simulink model "RudderActuatorChannel_control_arx"  (R2015a)
settings: Solver=ode4  StartTime=0.0  StopTime=2.999  FixedStep=sampleTime  MaxStep=1e-3  MinStep=1e-4
undefined symbols (not defined in the file or in its folder): Acv, Aleak1, Aleak2, Aleak3, Aleak4, Aleak5, Aleakext, Aleakint, Ap, Ap_seal, Ar_seal, As_ehsv, Bkp_seal, Bp1, C, Cd, ControlTopology, DeltaQ_ehsv, EHSV, EHSV_Step, EHSVFreqTest, EHSVTest, ent_air, frictionstribeck_velocity, i_ehsv, Imax, K2_ehsv, K3_ehsv, K_Supply1, Ka1, Kd, Ki, Ki_ehsv, Kp, Kr_ehsv, ksi_ehsv, Kst, Kst_Enable, Kw_ehsv, L0, Load_cmd, Lp_seal, Lr_seal, Max_Cmd, Max_Load_TED, Max_Load_TEU, Min_Cmd, Mp1, ON_OFF_hyst, P10, Pcvac, Pcvi, Pcvr, Ps0, Pt0, Ql_ehsv, R, Rate_Limit, Return_Pressure, Rho ... (+24)
undefined symbols (not defined in the file): dpLVDT, Kd_N, ramLVDT, StateControl, xvLVDT
libraries: simulink x3
(part 1 of 2)
settings Model: SimulationMode=accelerator  Creator=Charles  LastModifiedBy=Pedro H
settings SolverCC: InitialStep=1e-4
settings DataIOCC: LimitDataPoints=off  SaveFormat=StructureWithTime  DSMLogging=off  SaveTime=off
settings OptimizationCC: ExpressionDepthLimit=2147483647  InitFltsAndDblsToZero=on
settings DebuggingCC: SaveWithParameterizedLinksMsg=none  UnderspecifiedInitializationDetection=Classic  MergeDetectMultiDrivingBlocksExec=none  SolverPrmCheckMsg=warning  InheritedTsInSrcMsg=none  FcnCallInpInsideContextMsg=UseLocalSettings  StateNameClashWarn=warning
settings ModelReferenceCC: UpdateModelReferenceTargets=IfOutOfDate
settings GRTTargetCC: TargetFcnLib=ansi_tfl_tmw.mat  CombineOutputUpdateFcns=off  GRTInterface=on

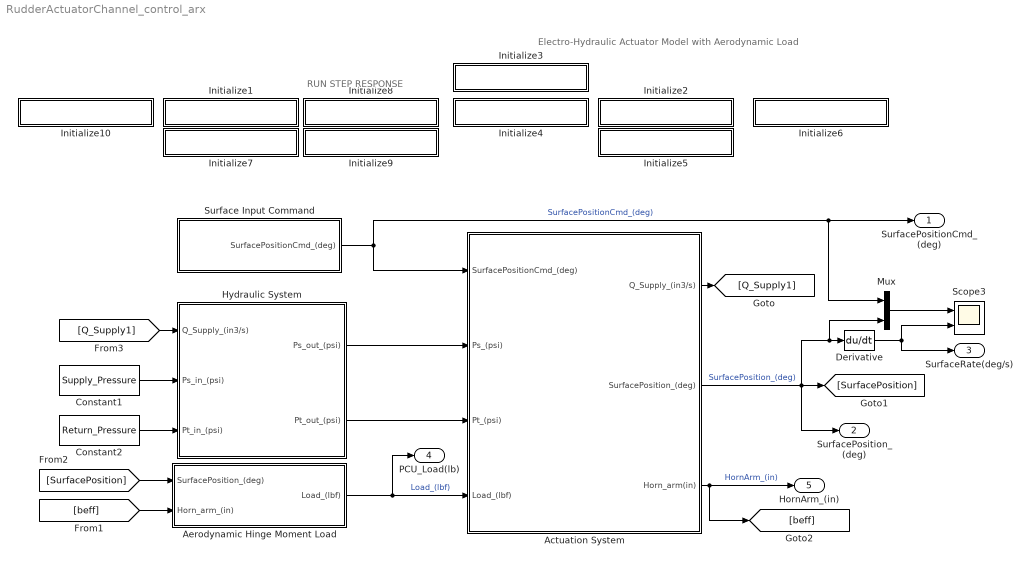
== system RudderActuatorChannel_control_arx ==
  note: RUN STEP RESPONSE
  note: Electro-Hydraulic Actuator Model with Aerodynamic Load
  Actuation System : Subsystem
  Aerodynamic Hinge Moment Load : Subsystem
  Constant1 : Constant  Value=Supply_Pressure
  Constant2 : Constant  Value=Return_Pressure
  Derivative : Derivative  CoefficientInTFapproximation=1e6
  Hydraulic System : Subsystem
  Initialize1 : Subsystem
      settings: OpenFcn=|
      | run('StepInput_CLLoad.m'),
      | set_param(bdroot,'SimulationCommand','start')
      mask Display: disp('Closed Loop - Loaded')
  Initialize10 : Subsystem
      settings: OpenFcn=|
      | run('SineInput_CLLoad.m'),
      | set_param(bdroot,'SimulationCommand','start')
      mask Display: disp('Run Sine Input')
  Initialize2 : Subsystem
      settings: OpenFcn=|
      | FreqResp_type = 0;
      | run('FrequencyResponseTest.m'),
      | set_param(bdroot,'SimulationCommand','start')
      mask Display: disp('Frequency Response')
  Initialize3 : Subsystem
      settings: OpenFcn=run('Load_Parameters.m'),
      mask Display: disp('Model Initialization')
  Initialize4 : Subsystem
      settings: OpenFcn=run('plotMaster.m')
      mask Display: disp('Plot Results')
  Initialize5 : Subsystem
      settings: OpenFcn=|
      | FreqResp_type = 1;
      | run('FrequencyResponseTest.m'),
      | set_param(bdroot,'SimulationCommand','start')
      mask Display: disp('Run EHSV Frequency Response Test')
  Initialize6 : Subsystem
      settings: OpenFcn=run('DynamicStiffnessTest.m')
      mask Display: disp('Dynamic Stiffness Test')
  Initialize7 : Subsystem
      settings: OpenFcn=|
      | run('StepInput_CLNoLoad.m'),
      | set_param(bdroot,'SimulationCommand','start')
      mask Display: disp('Closed Loop - Unloaded')
  Initialize8 : Subsystem
      settings: OpenFcn=|
      | run('StepInput_OLEHSVLoad.m'),
      | set_param(bdroot,'SimulationCommand','start')
      mask Display: disp('Open Loop - Loaded')
  Initialize9 : Subsystem
      settings: OpenFcn=|
      | run('StepInput_OLEHSVNoLoad.m'),
      | set_param(bdroot,'SimulationCommand','start')
      mask Display: disp('Open Loop - Unloaded')
  Mux : Mux  Inputs=2
  Scope3 : Scope  NumInputPorts=2
      settings: TimeRange=3.4  YMin=28.7~-5  YMax=30.8~5  SaveName=Theta
  Surface Input Command : Subsystem
  SurfacePositionCmd_(deg) : Outport
  SurfacePosition_(deg) : Outport  Port=2
  SurfaceRate(deg/s) : Outport  Port=3
  PCU_Load(lb) : Outport  Port=4
  HornArm_(in) : Outport  Port=5
  wires:
  Constant1/1 -> Hydraulic System/2(Ps_in_(psi))
  Constant2/1 -> Hydraulic System/3(Pt_in_(psi))
  Hydraulic System/1(Ps_out_(psi)) -> Actuation System/2(Ps_(psi))
  Hydraulic System/2(Pt_out_(psi)) -> Actuation System/3(Pt_(psi))
  Actuation System/1(Q_Supply_(in3/s)) -> [Q_Supply1]
  [Q_Supply1] -> Hydraulic System/1(Q_Supply_(in3/s))
  Actuation System/2(SurfacePosition_(deg)) -> SurfacePosition_(deg)/1, [SurfacePosition], Mux/2, Derivative/1  "SurfacePosition_(deg)"
  [SurfacePosition] -> Aerodynamic Hinge Moment Load/1(SurfacePosition_(deg))
  Surface Input Command/1(SurfacePositionCmd_(deg)) -> Mux/1, SurfacePositionCmd_(deg)/1, Actuation System/1(SurfacePositionCmd_(deg))  "SurfacePositionCmd_(deg)"
  Actuation System/3(Horn_arm(in)) -> [beff], HornArm_(in)/1  "HornArm_(in)"
  [beff] -> Aerodynamic Hinge Moment Load/2(Horn_arm_(in))
  Aerodynamic Hinge Moment Load/1(Load_(lbf)) -> Actuation System/4(Load_(lbf)), PCU_Load(lb)/1  "Load_(lbf)"
  Derivative/1 -> Scope3/2, SurfaceRate(deg/s)/1
  Mux/1 -> Scope3/1

== system RudderActuatorChannel_control_arx/Actuation System ==
  SurfacePositionCmd_(deg) : Inport
  Ps_(psi) : Inport  Port=2
  Pt_(psi) : Inport  Port=3
  Load_(lbf) : Inport  Port=4
  Actuator : Subsystem
  Bus Creator : BusCreator  Inputs=2
  Electronics System : Subsystem
  Scope : Scope
      settings: SaveName=ScopeData6
  Surface Kinematics : Subsystem
  Q_Supply_(in3/s) : Outport
  SurfacePosition_(deg) : Outport  Port=2
  Horn_arm(in) : Outport  Port=3
  wires:
  [Sensors_FB] -> Electronics System/2(Sensors_FB)
  SurfacePositionCmd_(deg)/1 -> [Theta_Cmd]
  [Theta_Cmd] -> Electronics System/1(Theta_Cmd_(deg))
  Ps_(psi)/1 -> Bus Creator/1  "Ps"
  Pt_(psi)/1 -> Bus Creator/2  "Pt"
  Bus Creator/1 -> Actuator/3(Hyd_Power)
  Actuator/2(Q_Supply) -> Q_Supply_(in3/s)/1
  Actuator/1(Xp_real_(in)) -> Surface Kinematics/1(Xp_(in))  "Xp"
  Load_(lbf)/1 -> [Load]
  Surface Kinematics/1(ThetaPos_(deg)) -> SurfacePosition_(deg)/1
  Actuator/3(Sensors) -> [Sensors_FB]
  Surface Kinematics/2(Effective_arm_(in)) -> Horn_arm(in)/1
  [Load] -> Scope/1, Actuator/2(Load)
  Electronics System/1(Current_Cmd_(mA)) -> Actuator/1(Current_Cmd)

== system RudderActuatorChannel_control_arx/Aerodynamic Hinge Moment Load ==
  note: Aerodynamic Hinge Moment Load
  SurfacePosition_(deg) : Inport
  Horn_arm_(in) : Inport  Port=2
  1-D Lookup Table : Lookup_n-D  NumberOfTableDimensions=1  BreakpointsForDimension1=[-1 0 1]  Table=[-Max_Load_TED 0 Max_Load_TEU]  RndMeth=Simplest  InputSameDT=on
  Constant : Constant  Value=StiffnessTest_Enable
  Constant1 : Constant  Value=Load_cmd
  Divide : Product  Inputs=*/
  Gain : Gain  Gain=1/Max_Cmd
  Load Type Selector : MultiPortSwitch
  Stiffness Test Load : Sin  Amplitude=StiffTest.Sine_Amplitude  Bias=StiffTest.Sine_Bias  Frequency=StiffTest.Sine_Frequency  SampleTime=0
  Load_(lbf) : Outport
  wires:
  SurfacePosition_(deg)/1 -> Gain/1
  Constant/1 -> Load Type Selector/1
  Gain/1 -> 1-D Lookup Table/1
  Load Type Selector/1 -> Load_(lbf)/1
  Stiffness Test Load/1 -> Load Type Selector/2
  Constant1/1 -> Load Type Selector/4
  1-D Lookup Table/1 -> Divide/1
  Divide/1 -> Load Type Selector/3
  Horn_arm_(in)/1 -> Divide/2

== system RudderActuatorChannel_control_arx/Hydraulic System ==
  Q_Supply_(in3/s) : Inport
  Ps_in_(psi) : Inport  Port=2
  Pt_in_(psi) : Inport  Port=3
  Aircraft Hydraulic Losses : Gain  Gain=K_Supply1
  Bus Selector : BusSelector  OutputSignals=Qs
  Fluid Inertia : TransferFcn  Denominator=[0.01 1]
  Sum1 : Sum  Inputs=|+-
  cis to gpm : Gain  Gain=0.25974
  Ps_out_(psi) : Outport
  Pt_out_(psi) : Outport  Port=2
  wires:
  Sum1/1 -> Ps_out_(psi)/1  "Ps"
  Aircraft Hydraulic Losses/1 -> Fluid Inertia/1
  Fluid Inertia/1 -> Sum1/2
  Pt_in_(psi)/1 -> Pt_out_(psi)/1  "Pt"
  Ps_in_(psi)/1 -> Sum1/1  "Ps"
  Q_Supply_(in3/s)/1 -> Bus Selector/1
  cis to gpm/1 -> Aircraft Hydraulic Losses/1
  Bus Selector/1 -> cis to gpm/1  "<Qs>"

== system RudderActuatorChannel_control_arx/Initialize1 ==

== system RudderActuatorChannel_control_arx/Initialize10 ==

== system RudderActuatorChannel_control_arx/Initialize2 ==

== system RudderActuatorChannel_control_arx/Initialize3 ==

== system RudderActuatorChannel_control_arx/Initialize4 ==

== system RudderActuatorChannel_control_arx/Initialize5 ==

== system RudderActuatorChannel_control_arx/Initialize6 ==

== system RudderActuatorChannel_control_arx/Initialize7 ==

== system RudderActuatorChannel_control_arx/Initialize8 ==

== system RudderActuatorChannel_control_arx/Initialize9 ==

== system RudderActuatorChannel_control_arx/Surface Input Command ==
  Repeating Sequence : simulink/Sources/Repeating Sequence  rep_seq_t=[0 0.001 1.5 1.501 3 3.001 4.5 4.501 6 6.001 7.5 7.501 9 9.001 10.5 10.501 12 12.001 13.5 13.501 15]  rep_seq_y=[0 1 1 -1 -1 0.6 0.6 -0.8 -0.8 -0.1 -0.1 0.9 0.9 -0.7 -0.7 0 0 -0.5 -0.5 1 1]
  Repeating Sequence1 : simulink/Sources/Repeating Sequence  rep_seq_t=[0 0.001 1 1.001 2 2.001 3 3.001 4 4.001 5 5.001 6 6.001 7 7.001 8 8.001 9 9.001 10 10.001 11 11.001 12 12.001 13 13.001 14 14.001 15]  rep_seq_y=[0 1 1 1 1 -1 -1 1 1 -1 -1 -1 -1 1 1 1 1 -1 -1 1 1 -1 -1 -1 -1 -1 -1 1 1 1 1]
  SurfacePositionCmd_(deg) : Outport
  wires:
  Repeating Sequence/1 -> SurfacePositionCmd_(deg)/1

== system RudderActuatorChannel_control_arx/Actuation System/Actuator ==
  Current_Cmd : Inport
  Load : Inport  Port=2
  Hyd_Power : Inport  Port=3
  Cylinder Dynamics : Subsystem
  Sensors Dynamics : Subsystem
  Valves Dynamics : Subsystem
  Xp_real_(in) : Outport
  Q_Supply : Outport  Port=2
  Sensors : Outport  Port=3
  wires:
  Cylinder Dynamics/2(Xp) -> [Xp], Xp_real_(in)/1
  Load/1 -> Cylinder Dynamics/2(Load)
  Valves Dynamics/2(Q_Supply) -> Q_Supply/1
  Valves Dynamics/1(Q_Act) -> Cylinder Dynamics/1(Q_Act)
  Current_Cmd/1 -> Valves Dynamics/2(Currrent)
  Hyd_Power/1 -> Valves Dynamics/3(Hyd_Pwr)
  Cylinder Dynamics/1(P_Act) -> Valves Dynamics/1(P_Act)
  Cylinder Dynamics/3(Qacv) -> Valves Dynamics/4(Qacv)
  Valves Dynamics/3(Pt) -> Cylinder Dynamics/3(Pt)
  Valves Dynamics/4(Xv_(in)) -> [Xv]
  Cylinder Dynamics/4(dP) -> [dP]
  [Xp] -> Sensors Dynamics/1(Xp)
  [dP] -> Sensors Dynamics/2(dP)
  [Xv] -> Sensors Dynamics/3(Xv)
  Sensors Dynamics/1(Sensors) -> Sensors/1

== system RudderActuatorChannel_control_arx/Actuation System/Electronics System ==
  Theta_Cmd_(deg) : Inport
  Sensors_FB : Inport  Port=2
  Analog Controller : Subsystem
  Constant : Constant  Value=ControlTopology
  Digital Controller : Subsystem
  Hardware_in : Subsystem
  Hardware_out : Subsystem
  Switch : Switch  Threshold=5.5
  Current_Cmd_(mA) : Outport
  wires:
  Theta_Cmd_(deg)/1 -> Analog Controller/1(Cmd_D), Hardware_in/1(Theta_Cmd_in)
  Digital Controller/1(EHSV_Cmd) -> Hardware_out/1(EHSV_Cmd_in)
  Hardware_out/1(EHSV_Cmd_out) -> Switch/3  "Current_Cmd_CL"
  Hardware_in/1(Theta_Cmd_out) -> Digital Controller/1(Cmd_D)
  Hardware_in/2(Sensors_FB_out) -> Digital Controller/2(Sensors_FB)
  Sensors_FB/1 -> Analog Controller/2(Sensors_FB), Hardware_in/2(Sensors_FB_in)
  Switch/1 -> Current_Cmd_(mA)/1
  Analog Controller/1(EHSV_Cmd) -> Switch/1
  Constant/1 -> Switch/2

== system RudderActuatorChannel_control_arx/Actuation System/Surface Kinematics ==
  Xp_(in) : Inport
  Rad2Deg : Gain  Gain=180/pi  SaturateOnIntegerOverflow=on  OutDataTypeStr=Inherit: Same as input  ParamDataTypeStr=Inherit: Same as input
  Real Kinematics : Subsystem
  ThetaPos_(deg) : Outport
  Effective_arm_(in) : Outport  Port=2
  wires:
  Xp_(in)/1 -> Real Kinematics/1(Xp)
  Real Kinematics/1(Theta) -> Rad2Deg/1
  Rad2Deg/1 -> ThetaPos_(deg)/1
  Real Kinematics/2(Reff) -> Effective_arm_(in)/1

== system RudderActuatorChannel_control_arx/Actuation System/Actuator/Cylinder Dynamics ==
  Q_Act : Inport
  Load : Inport  Port=2
  Pt : Inport  Port=3
  Bus Creator1 : BusCreator  Inputs=2
  Bus Creator3 : BusCreator  Inputs=2
  Bus Selector : BusSelector  OutputSignals=Q1,Q2
  Fluid Dynamics : Subsystem
  Piston Dynamics : Subsystem
  Scope : Scope  NumInputPorts=5
      settings: YMin=-5~-5~-5~-5~-5  YMax=5~5~5~5~5  SaveName=ScopeData8
  P_Act : Outport
  Xp : Outport  Port=2
  Qacv : Outport  Port=3
  dP : Outport  Port=4
  wires:
  Bus Creator3/1 -> P_Act/1
  Q_Act/1 -> Bus Selector/1
  Bus Selector/2 -> Fluid Dynamics/4(Q2)  "<Q2>"
  Piston Dynamics/1(Xp) -> [Xp], Xp/1
  Piston Dynamics/2(Xpdot) -> [Xpdot]  "Xpdot"
  [Xp] -> Scope/3, Fluid Dynamics/1(xp)
  [Xpdot] -> Scope/4, Fluid Dynamics/2(xpdot)
  Load/1 -> Piston Dynamics/3(FL)
  Bus Selector/1 -> Fluid Dynamics/3(Q1)  "<Q1>"
  Fluid Dynamics/2(P2) -> Scope/2, Piston Dynamics/2(Pr), Bus Creator3/2  "P2"
  Fluid Dynamics/1(P1) -> Scope/1, Piston Dynamics/1(Pe), Bus Creator3/1  "P1"
  Pt/1 -> Fluid Dynamics/5(Pt)
  Fluid Dynamics/3(Qacv1) -> Bus Creator1/1  "Qacv1"
  Fluid Dynamics/4(Qacv2) -> Bus Creator1/2  "Qacv2"
  Bus Creator1/1 -> Qacv/1
  Fluid Dynamics/5(dP) -> Scope/5, dP/1

== system RudderActuatorChannel_control_arx/Actuation System/Actuator/Sensors Dynamics ==
  Xp : Inport
  dP : Inport  Port=2
  Xv : Inport  Port=3
  Bus Creator : BusCreator  Inputs=3
  "Xp LVDT " : Subsystem
  "Xv LVDT " : Subsystem
  "dP LVDT " : Subsystem
  Sensors : Outport
  wires:
  dP/1 -> "dP LVDT "/1(dP_real)
  Xp/1 -> "Xp LVDT "/1(Xp_real)
  Xv/1 -> "Xv LVDT "/1(Xv_real)
  "Xv LVDT "/1(Xv_LVDT) -> Bus Creator/3  "Xv_mesured_(in)"
  "dP LVDT "/1(dP_LVDT) -> Bus Creator/2  "dP_mesured_(psi)"
  "Xp LVDT "/1(Xp_LVDT) -> Bus Creator/1  "Xp_mesured_(in)"
  Bus Creator/1 -> Sensors/1

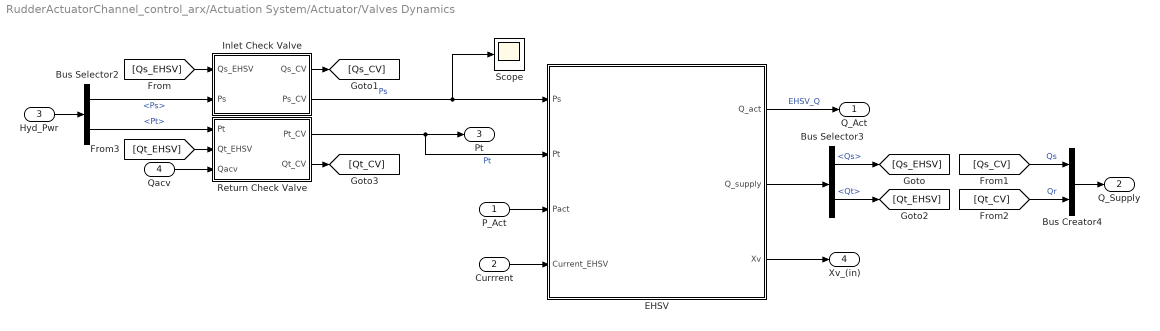
== system RudderActuatorChannel_control_arx/Actuation System/Actuator/Valves Dynamics ==
  P_Act : Inport
  Currrent : Inport  Port=2
  Hyd_Pwr : Inport  Port=3
  Qacv : Inport  Port=4
  Bus Creator4 : BusCreator  Inputs=2
  Bus Selector2 : BusSelector  OutputSignals=Ps,Pt
  Bus Selector3 : BusSelector  OutputSignals=Qs,Qt
  EHSV : Subsystem
  Inlet Check Valve : Subsystem
  Return Check Valve : Subsystem
  Scope : Scope
      settings: SaveName=ScopeData5
  Q_Act : Outport
  Q_Supply : Outport  Port=2
  Pt : Outport  Port=3
  Xv_(in) : Outport  Port=4
  wires:
  Hyd_Pwr/1 -> Bus Selector2/1
  EHSV/1(Q_act) -> Q_Act/1  "EHSV_Q"
  Bus Selector2/1 -> Inlet Check Valve/2(Ps)  "<Ps>"
  Bus Selector3/1 -> [Qs_EHSV]  "<Qs>"
  [Qs_EHSV] -> Inlet Check Valve/1(Qs_EHSV)
  Inlet Check Valve/1(Qs_CV) -> [Qs_CV]
  [Qs_CV] -> Bus Creator4/1  "Qs"
  Bus Creator4/1 -> Q_Supply/1
  Bus Selector2/2 -> Return Check Valve/1(Pt)  "<Pt>"
  Bus Selector3/2 -> [Qt_EHSV]  "<Qt>"
  [Qt_CV] -> Bus Creator4/2  "Qr"
  [Qt_EHSV] -> Return Check Valve/2(Qt_EHSV)
  Return Check Valve/2(Qt_CV) -> [Qt_CV]
  Qacv/1 -> Return Check Valve/3(Qacv)
  Currrent/1 -> EHSV/4(Current_EHSV)
  P_Act/1 -> EHSV/3(Pact)
  Inlet Check Valve/2(Ps_CV) -> Scope/1, EHSV/1(Ps)  "Ps"
  Return Check Valve/1(Pt_CV) -> EHSV/2(Pt), Pt/1  "Pt"
  EHSV/2(Q_supply) -> Bus Selector3/1
  EHSV/3(Xv) -> Xv_(in)/1

== system RudderActuatorChannel_control_arx/Actuation System/Electronics System/Analog Controller ==
  Cmd_D : Inport
  Sensors_FB : Inport  Port=2
  Command Limits : Saturate  UpperLimit=Max_Cmd  LowerLimit=Min_Cmd
  Deg2Rad : Gain  Gain=pi/180  SaturateOnIntegerOverflow=on  OutDataTypeStr=Inherit: Same as input  ParamDataTypeStr=Inherit: Same as input
  Demux : Demux  Outputs=3
  Kinematics : Subsystem
  LQR : Subsystem  mask{K=[14.6507   -0.0011   -0.0000    0.0003   22.9112   -0.0053]}
      mask prompts: K "State Control gain (K)"
  Mux : Mux  Inputs=3
  Rate Limiter : RateLimiter  RisingSlewLimit=Rate_Limit*0.9  FallingSlewLimit=-Rate_Limit*0.9  SampleTimeMode=inherited
  Reduced order observer : Subsystem  mask{H=StateControl.Obs.H, A=StateControl.Obs.A, K=StateControl.Obs.K, L=StateControl.Obs.L}
      mask prompts: H "H obs"; A "A obs"; K "K obs"; L "L obs"
  Saturation +/- 10mA : Saturate  UpperLimit=Imax  LowerLimit=-Imax
  Scope : Scope
      settings: TimeRange=3  YMin=0  YMax=3.5  SaveName=ScopeData9
  Scope1 : Scope  NumInputPorts=2
      settings: YMin=-5~-5  YMax=5~5  SaveName=ScopeData10
  Scope2 : Scope  NumInputPorts=3
      settings: YMin=-5~-5~-5  YMax=5~5~5  SaveName=ScopeData11
  Sgn Convention : Gain  SaturateOnIntegerOverflow=on  OutDataTypeStr=Inherit: Same as input  ParamDataTypeStr=Inherit: Same as input
  To Workspace : ToWorkspace  VariableName=simout  SaveFormat=Timeseries  SampleTime=-1
  EHSV_Cmd : Outport
  wires:
  Cmd_D/1 -> Rate Limiter/1
  Kinematics/1(Xp) -> Scope/1, LQR/1(Ref)  "Pos_Cmd"
  Command Limits/1 -> Sgn Convention/1
  Deg2Rad/1 -> Kinematics/1(ThetaS)
  Rate Limiter/1 -> Command Limits/1
  Sgn Convention/1 -> Deg2Rad/1
  Sensors_FB/1 -> Demux/1
  Demux/1 -> Scope2/1, Mux/3  "<Xp_FB>"
  Demux/2 -> Scope2/2, Mux/2, To Workspace/1  "<dP_FB>"
  Demux/3 -> Scope2/3, Mux/1  "<Xv_FB>"
  Mux/1 -> Reduced order observer/1(y)
  Reduced order observer/1(Xobs) -> LQR/2(Xobs)
  LQR/1(u) -> Scope1/1, Saturation +/- 10mA/1
  Saturation +/- 10mA/1 -> Reduced order observer/2(u), Scope1/2, EHSV_Cmd/1

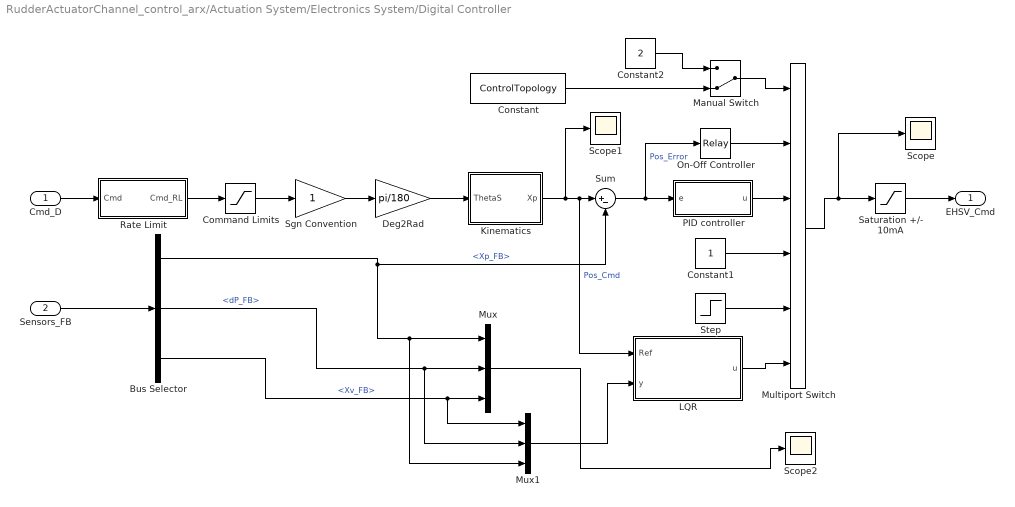
== system RudderActuatorChannel_control_arx/Actuation System/Electronics System/Digital Controller ==
  Cmd_D : Inport
  Sensors_FB : Inport  Port=2
  Bus Selector : BusSelector  OutputSignals=Xp_FB,dP_FB,Xv_FB
  Command Limits : Saturate  UpperLimit=Max_Cmd  LowerLimit=Min_Cmd
  Constant : Constant  Value=ControlTopology
  Constant1 : Constant
  Constant2 : Constant  Value=2
  Deg2Rad : Gain  Gain=pi/180  SampleTime=T_ES  SaturateOnIntegerOverflow=on  OutDataTypeStr=Inherit: Same as input  ParamDataTypeStr=Inherit: Same as input
  Kinematics : Subsystem
  LQR : Subsystem  mask{K=[14.6507 0.0003   22.9112 ]}
      mask prompts: K "State Control gain (K)"
  Manual Switch : ManualSwitch  CurrentSetting=0
  Multiport Switch : MultiPortSwitch  Inputs=5
  Mux : Mux  Inputs=3
  Mux1 : Mux  Inputs=3
  On-Off Controller : Relay  OnSwitchValue=ON_OFF_hyst  OffSwitchValue=-ON_OFF_hyst  OnOutputValue=10  OffOutputValue=-10
  PID controller : Subsystem  mask{Kp=Kp, Ki=Ki, Kd=Kd, Ts=T_ES, kd_N=Kd_N, umax=10}
      mask prompts: Ts "Sampling Time"; kd_N "Kd Filter coefficient"; umax "Max command"
  Rate Limit : Subsystem
  Saturation +/- 10mA : Saturate  UpperLimit=Imax  LowerLimit=-Imax  SampleTime=T_ES
  Scope : Scope
  Scope1 : Scope
      settings: SaveName=ScopeData2
  Scope2 : Scope
      settings: SaveName=ScopeData7
  Sgn Convention : Gain  SampleTime=T_ES  SaturateOnIntegerOverflow=on  OutDataTypeStr=Inherit: Same as input  ParamDataTypeStr=Inherit: Same as input
  Step : Step  Time=EHSV_Step.time  Before=EHSV_Step.initial  After=EHSV_Step.final
  Sum : Sum  Inputs=|+-  SampleTime=T_ES  SaturateOnIntegerOverflow=on  InputSameDT=on  OutDataTypeStr=Inherit: Same as first input
  EHSV_Cmd : Outport
  wires:
  Cmd_D/1 -> Rate Limit/1(Cmd)
  Kinematics/1(Xp) -> Scope1/1, LQR/1(Ref), Sum/1  "Pos_Cmd"
  Saturation +/- 10mA/1 -> EHSV_Cmd/1
  Sum/1 -> On-Off Controller/1, PID controller/1(e)  "Pos_Error"
  Command Limits/1 -> Sgn Convention/1
  Deg2Rad/1 -> Kinematics/1(ThetaS)
  Rate Limit/1(Cmd_RL) -> Command Limits/1
  Sgn Convention/1 -> Deg2Rad/1
  Sensors_FB/1 -> Bus Selector/1
  Bus Selector/1 -> Sum/2, Mux1/3, Mux/1  "<Xp_FB>"
  Bus Selector/2 -> Mux1/2, Mux/2  "<dP_FB>"
  Bus Selector/3 -> Mux1/1, Mux/3  "<Xv_FB>"
  Multiport Switch/1 -> Scope/1, Saturation +/- 10mA/1
  Constant/1 -> Manual Switch/2
  On-Off Controller/1 -> Multiport Switch/2
  Constant1/1 -> Multiport Switch/4
  PID controller/1(u) -> Multiport Switch/3
  Step/1 -> Multiport Switch/5
  Mux/1 -> Scope2/1
  Manual Switch/1 -> Multiport Switch/1
  Constant2/1 -> Manual Switch/1
  Mux1/1 -> LQR/2(y)
  LQR/1(u) -> Multiport Switch/6

== system RudderActuatorChannel_control_arx/Actuation System/Electronics System/Hardware_in ==
  Theta_Cmd_in : Inport
  Sensors_FB_in : Inport  Port=2
  Bus Creator : BusCreator  Inputs=3
  Bus Selector : BusSelector  OutputSignals=Xp_FB,dP_FB,Xv_FB
  Rate Transition{2..5} (4 alike) : RateTransition  Deterministic=off  OutPortSampleTime=T_ES
  Signal Processing : Subsystem
  Theta_Cmd_out : Outport
  Sensors_FB_out : Outport  Port=2
  wires:
  Bus Creator/1 -> Sensors_FB_out/1
  Theta_Cmd_in/1 -> Rate Transition2/1
  Rate Transition2/1 -> Theta_Cmd_out/1
  Sensors_FB_in/1 -> Signal Processing/1(Sesnsors_In)
  Bus Selector/1 -> Rate Transition3/1  "<Xp_FB>"
  Rate Transition3/1 -> Bus Creator/1  "Xp_FB"
  Rate Transition4/1 -> Bus Creator/2  "dP_FB"
  Rate Transition5/1 -> Bus Creator/3  "Xv_FB"
  Bus Selector/2 -> Rate Transition4/1  "<dP_FB>"
  Bus Selector/3 -> Rate Transition5/1  "<Xv_FB>"
  Signal Processing/1(Sensors_Out) -> Bus Selector/1

== system RudderActuatorChannel_control_arx/Actuation System/Electronics System/Hardware_out ==
  EHSV_Cmd_in : Inport
  Rate Transition : RateTransition  Deterministic=off  OutPortSampleTime=0
  Servoamplifier Dynamics : TransferFcn  Numerator=[100]  Denominator=[1 100]
  Servoamplifier Tolerance : Gain  Gain=Tol_SA1
  EHSV_Cmd_out : Outport
  wires:
  Rate Transition/1 -> Servoamplifier Dynamics/1
  Servoamplifier Dynamics/1 -> Servoamplifier Tolerance/1
  EHSV_Cmd_in/1 -> Rate Transition/1
  Servoamplifier Tolerance/1 -> EHSV_Cmd_out/1  "Current"

== system RudderActuatorChannel_control_arx/Actuation System/Surface Kinematics/Real Kinematics ==
  Xp : Inport
  Bus Creator : BusCreator
  Bus Selector2 : BusSelector  OutputSignals=C,R,L
  Bus Selector3 : BusSelector  OutputSignals=L,C,R
  Bus Selector4 : BusSelector  OutputSignals=Theta0
  Bus Selector5 : BusSelector  OutputSignals=C
  Constant : Constant  Value=L0
  Constant1 : Constant  Value=R
  Constant2 : Constant  Value=C
  Constant3 : Constant  Value=Theta0
  Law of cosines Get angle : Fcn  Expr=acos((u(1)^2+u(2)^2-u(3)^2)/(2*u(1)*u(2)))
  Law of cosines Get angle1 : Fcn  Expr=acos((u(1)^2+u(2)^2-u(3)^2)/(2*u(1)*u(2)))
  Mux1 : Mux  Inputs=3
  Mux2 : Mux  Inputs=3
  Product : Product  RndMeth=Zero
  Sum1 : Sum  Inputs=++|
  Sum4 : Sum  Inputs=|+-
  Trigonometric Function : Trigonometry
  Theta : Outport
  Reff : Outport  Port=2
  wires:
  Mux2/1 -> Law of cosines Get angle1/1
  Bus Selector2/1 -> Mux2/1  "<C>"
  Bus Selector2/2 -> Mux2/2  "<R>"
  Law of cosines Get angle1/1 -> Sum4/1  "theta"
  Bus Selector4/1 -> Sum4/2  "<Theta0>"
  Sum4/1 -> Theta/1
  Xp/1 -> Sum1/1  "Xp"
  Constant/1 -> Sum1/2  "L0"
  Sum1/1 -> Bus Creator/1  "L"
  Constant2/1 -> Bus Creator/2  "C"
  Constant1/1 -> Bus Creator/3  "R"
  Constant3/1 -> Bus Creator/4  "Theta0"
  Mux1/1 -> Law of cosines Get angle/1
  Law of cosines Get angle/1 -> Trigonometric Function/1  "alfa"
  Bus Selector3/1 -> Mux1/1  "<L>"
  Bus Selector3/2 -> Mux1/2  "<C>"
  Bus Selector3/3 -> Mux1/3  "<R>"
  Product/1 -> Reff/1  "Reff"
  Bus Selector5/1 -> Product/1  "<C>"
  Trigonometric Function/1 -> Product/2
  Bus Selector2/3 -> Mux2/3  "<L>"
  Bus Creator/1 -> Bus Selector3/1, Bus Selector5/1, Bus Selector2/1, Bus Selector4/1

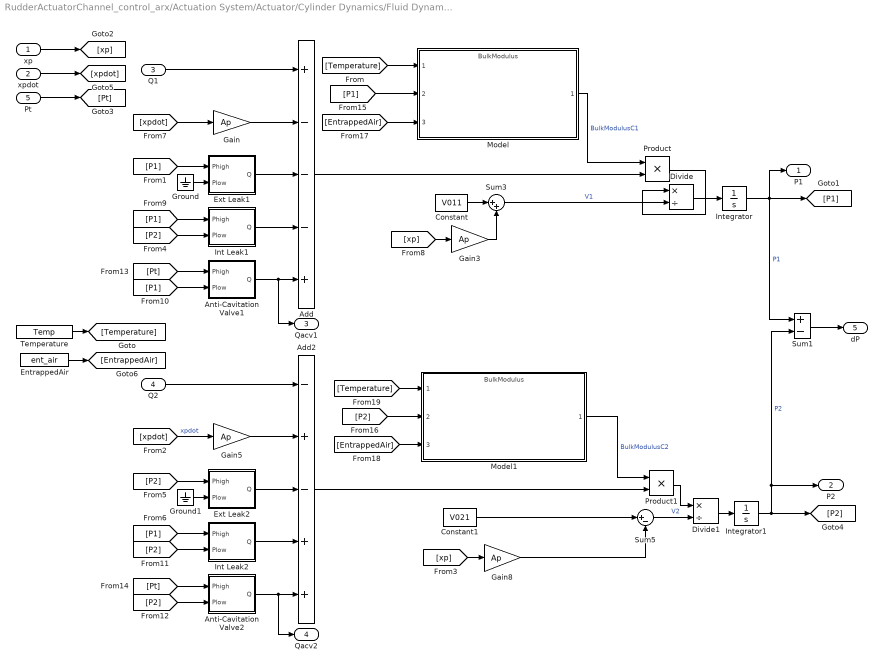
== system RudderActuatorChannel_control_arx/Actuation System/Actuator/Cylinder Dynamics/Fluid Dynamics ==
  xp : Inport
  xpdot : Inport  Port=2
  Q1 : Inport  Port=3
  Q2 : Inport  Port=4
  Pt : Inport  Port=5
  Add : Sum  Inputs=+---+
  Add2 : Sum  Inputs=-+-++
  Anti-Cavitation Valve1 : Subsystem
  Anti-Cavitation Valve2 : Subsystem
  Constant : Constant  Value=V011
  Constant1 : Constant  Value=V021
  Divide : Product  Inputs=*/
  Divide1 : Product  Inputs=*/
  EntrappedAir : Constant  Value=ent_air
  Ext Leak1 : Subsystem
  Ext Leak2 : Subsystem
  Gain{,3,5,8} (4 alike) : Gain  Gain=Ap
  Ground : Ground
  Ground1 : Ground
  Int Leak1 : Subsystem
  Int Leak2 : Subsystem
  Integrator : Integrator  InitialCondition=P10
  Integrator1 : Integrator  InitialCondition=P10
  Model : ModelReference  ModelNameDialog=BulkModulus  SimulationMode=Normal  ModelReferenceVersion=1.12  CopyOfModelName=BulkModulus  DefaultDataLogging=on
  Model1 : ModelReference  ModelNameDialog=BulkModulus  SimulationMode=Normal  ModelReferenceVersion=1.12  CopyOfModelName=BulkModulus  DefaultDataLogging=on
  Product : Product  RndMeth=Zero
  Product1 : Product  RndMeth=Zero
  Sum1 : Sum  Inputs=+-
  Sum3 : Sum  Inputs=|++
  Sum5 : Sum  Inputs=|+-
  Temperature : Constant  Value=Temp
  P1 : Outport
  P2 : Outport  Port=2
  Qacv1 : Outport  Port=3
  Qacv2 : Outport  Port=4
  dP : Outport  Port=5
  wires:
  Q1/1 -> Add/1
  Q2/1 -> Add2/1
  [xpdot] -> Gain5/1  "xpdot"
  [xp] -> Gain8/1
  Int Leak2/1(Q) -> Add2/4
  Divide1/1 -> Integrator1/1
  Sum5/1 -> Divide1/2  "V2"
  Gain8/1 -> Sum5/2
  Constant1/1 -> Sum5/1
  Integrator1/1 -> [P2], Sum1/2, P2/1  "P2"
  Ext Leak2/1(Q) -> Add2/3
  Gain5/1 -> Add2/2
  Int Leak1/1(Q) -> Add/4
  Divide/1 -> Integrator/1
  Sum3/1 -> Divide/2  "V1"
  Gain3/1 -> Sum3/2
  Constant/1 -> Sum3/1
  Integrator/1 -> Sum1/1, [P1], P1/1  "P1"
  Ext Leak1/1(Q) -> Add/3
  Add/1 -> Product/2
  Gain/1 -> Add/2
  [P1] -> Ext Leak1/1(Phigh)
  [P2] -> Ext Leak2/1(Phigh)
  xpdot/1 -> [xpdot]
  [xpdot] -> Gain/1
  xp/1 -> [xp]
  [xp] -> Gain3/1
  [P2] -> Int Leak1/2(Plow)
  Ground/1 -> Ext Leak1/2(Plow)
  Ground1/1 -> Ext Leak2/2(Plow)
  [P1] -> Int Leak2/1(Phigh)
  [Pt] -> Anti-Cavitation Valve1/1(Phigh)
  [P1] -> Anti-Cavitation Valve1/2(Plow)
  [P1] -> Int Leak1/1(Phigh)
  Anti-Cavitation Valve1/1(Q) -> Add/5, Qacv1/1
  [P2] -> Int Leak2/2(Plow)
  Anti-Cavitation Valve2/1(Q) -> Add2/5, Qacv2/1
  [Pt] -> Anti-Cavitation Valve2/1(Phigh)
  [P2] -> Anti-Cavitation Valve2/2(Plow)
  Pt/1 -> [Pt]
  Product/1 -> Divide/1
  [P1] -> Model/2
  Model/1 -> Product/1  "BulkModulusC1"
  Product1/1 -> Divide1/1
  Model1/1 -> Product1/1  "BulkModulusC2"
  Add2/1 -> Product1/2
  [P2] -> Model1/2
  Temperature/1 -> [Temperature]
  EntrappedAir/1 -> [EntrappedAir]
  [Temperature] -> Model/1
  [EntrappedAir] -> Model/3
  [EntrappedAir] -> Model1/3
  [Temperature] -> Model1/1
  Sum1/1 -> dP/1

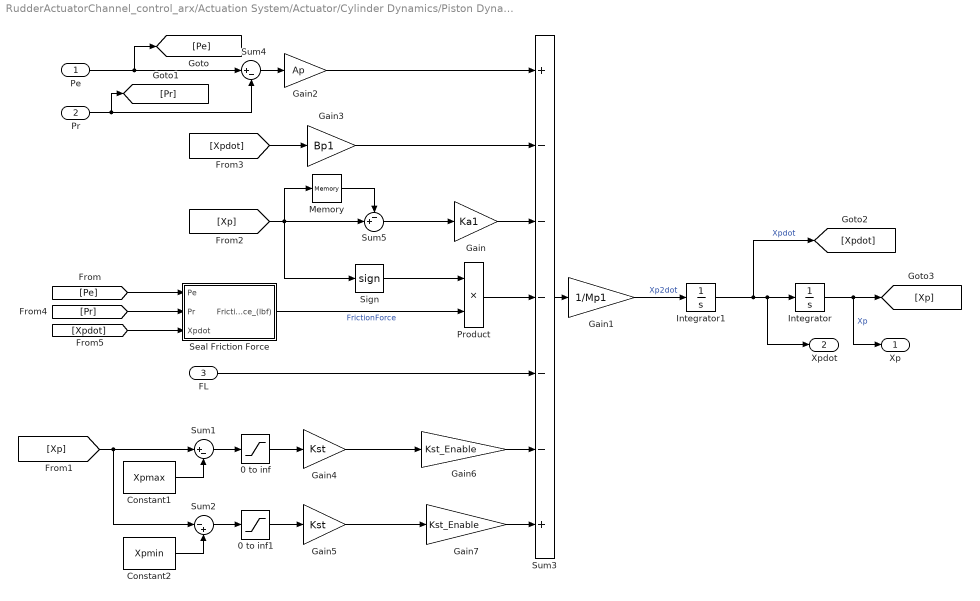
== system RudderActuatorChannel_control_arx/Actuation System/Actuator/Cylinder Dynamics/Piston Dynamics ==
  Pe : Inport
  Pr : Inport  Port=2
  FL : Inport  Port=3
  0 to inf : Saturate  UpperLimit=inf  LowerLimit=0
  0 to inf1 : Saturate  UpperLimit=inf  LowerLimit=0
  Constant1 : Constant  Value=Xpmax
  Constant2 : Constant  Value=Xpmin
  Gain : Gain  Gain=Ka1
  Gain1 : Gain  Gain=1/Mp1
  Gain2 : Gain  Gain=Ap
  Gain3 : Gain  Gain=Bp1
  Gain4 : Gain  Gain=Kst
  Gain5 : Gain  Gain=Kst
  Gain6 : Gain  Gain=Kst_Enable
  Gain7 : Gain  Gain=Kst_Enable
  Integrator : Integrator  InitialCondition=Xp_init
  Integrator1 : Integrator  InitialCondition=0.01
  Memory : Memory
  Product : Product  RndMeth=Zero
  Seal Friction Force : Subsystem
  Sign : Signum
  Sum1 : Sum  Inputs=|+-
  Sum2 : Sum  Inputs=|-+
  Sum3 : Sum  Inputs=+-----+
  Sum4 : Sum  Inputs=|+-
  Sum5 : Sum  Inputs=-+|
  Xp : Outport
  Xpdot : Outport  Port=2
  wires:
  Sum3/1 -> Gain1/1
  Gain1/1 -> Integrator1/1  "Xp2dot"
  Integrator1/1 -> Integrator/1, Xpdot/1, [Xpdot]  "Xpdot"
  Integrator/1 -> [Xp], Xp/1  "Xp"
  [Xp] -> Sign/1, Sum5/2, Memory/1
  Pe/1 -> [Pe], Sum4/1
  Sum4/1 -> Gain2/1
  Gain2/1 -> Sum3/1
  [Xpdot] -> Gain3/1
  Gain3/1 -> Sum3/2
  Gain/1 -> Sum3/3
  FL/1 -> Sum3/5
  Sum1/1 -> 0 to inf/1
  0 to inf/1 -> Gain4/1
  Constant2/1 -> Sum2/2
  Sign/1 -> Product/1
  Product/1 -> Sum3/4
  [Xp] -> Sum1/1, Sum2/1
  Gain4/1 -> Gain6/1
  Sum2/1 -> 0 to inf1/1
  0 to inf1/1 -> Gain5/1
  Gain5/1 -> Gain7/1
  Constant1/1 -> Sum1/2
  Memory/1 -> Sum5/1
  Sum5/1 -> Gain/1
  Seal Friction Force/1(FrictionForce_(lbf)) -> Product/2  "FrictionForce"
  Pr/1 -> [Pr], Sum4/2
  [Pr] -> Seal Friction Force/2(Pr)
  [Pe] -> Seal Friction Force/1(Pe)
  Gain6/1 -> Sum3/6
  Gain7/1 -> Sum3/7
  [Xpdot] -> Seal Friction Force/3(Xpdot)

== system RudderActuatorChannel_control_arx/Actuation System/Actuator/Sensors Dynamics/Xp LVDT  ==
  Xp_real : Inport
  LVDT : Subsystem  mask{band=ramLVDT.Bandwidth, range=ramLVDT.Range, lvdt_error=ramLVDT.Error, hyst=ramLVDT.Hysteresis}
      mask prompts: band "LVDT Bandwdidth"; range "LVDT Range ([min middle max])"; lvdt_error "LVDT error"; hyst "LVDT Hysteresis"
  Xp_LVDT : Outport
  wires:
  Xp_real/1 -> LVDT/1(Sensor In)
  LVDT/1(SensorOut) -> Xp_LVDT/1

== system RudderActuatorChannel_control_arx/Actuation System/Actuator/Sensors Dynamics/Xv LVDT  ==
  Xv_real : Inport
  LVDT1 : Subsystem  mask{band=xvLVDT.Bandwidth, range=xvLVDT.Range, lvdt_error=xvLVDT.Error, hyst=xvLVDT.Hysteresis}
      mask prompts: band "LVDT Bandwdidth (Hz)"; range "LVDT Range ([min middle max])"; lvdt_error "LVDT error"; hyst "LVDT Hysteresis (%)"
  Xv_LVDT : Outport
  wires:
  Xv_real/1 -> LVDT1/1(Sensor In)
  LVDT1/1(SensorOut) -> Xv_LVDT/1

== system RudderActuatorChannel_control_arx/Actuation System/Actuator/Sensors Dynamics/dP LVDT  ==
  dP_real : Inport
  LVDT1 : Subsystem  mask{band=dpLVDT.Bandwidth, range=dpLVDT.Range, lvdt_error=dpLVDT.Error, hyst=dpLVDT.Hysteresis}
      mask prompts: band "LVDT Bandwdidth (Hz)"; range "LVDT Range ([min middle max])"; lvdt_error "LVDT error"; hyst "LVDT Hysteresis (%)"
  dP_LVDT : Outport
  wires:
  dP_real/1 -> LVDT1/1(Sensor In)
  LVDT1/1(SensorOut) -> dP_LVDT/1

== system RudderActuatorChannel_control_arx/Actuation System/Actuator/Valves Dynamics/EHSV ==
  Ps : Inport
  Pt : Inport  Port=2
  Pact : Inport  Port=3
  Current_EHSV : Inport  Port=4
  Bus Selector1 : BusSelector  OutputSignals=P1,P2
  Derivative : Derivative
  EHSV 1st Stage : Subsystem
  EHSV 2nd Stage : Subsystem
  EHSV Test : Subsystem
  EHSV Test1 : Subsystem
  EHSV Test2 : Subsystem
  EHSV Test3 : Subsystem
  EHSV input : Subsystem
  Scope : Scope
  Scope1 : Scope  NumInputPorts=2
      settings: YMin=-5~-5  YMax=5~5  SaveName=ScopeData4
  Q_act : Outport
  Q_supply : Outport  Port=2
  Xv : Outport  Port=3
  wires:
  Bus Selector1/1 -> EHSV Test/1(In1)  "<P1>"
  Bus Selector1/2 -> EHSV Test1/1(In1)  "<P2>"
  EHSV 1st Stage/1(Xv) -> Derivative/1, Xv/1, EHSV 2nd Stage/5(Xv)  "Xv"
  EHSV Test/1(Out1) -> EHSV 2nd Stage/3(P1)  "P1"
  EHSV Test1/1(Out1) -> EHSV 2nd Stage/4(P2)  "P2"
  Pt/1 -> EHSV Test3/1(In1)
  EHSV 2nd Stage/1(Q) -> Q_act/1  "EHSV_Q"
  Ps/1 -> EHSV Test2/1(In1)
  Current_EHSV/1 -> EHSV input/1(CurrentCmd)
  Pact/1 -> Bus Selector1/1
  EHSV 2nd Stage/2(Q_Supply) -> Q_supply/1
  EHSV Test2/1(Out1) -> EHSV 2nd Stage/1(Ps)  "Ps"
  EHSV Test3/1(Out1) -> EHSV 2nd Stage/2(Pt)  "Pt"
  EHSV input/1(EHSV_current) -> EHSV 1st Stage/1(i)  "EHSV_current_cmd"
  EHSV 2nd Stage/3(Q_leak_EHV) -> Scope/1  "Qleak_EHSV"
  Derivative/1 -> Scope1/1, Scope1/2

== system RudderActuatorChannel_control_arx/Actuation System/Actuator/Valves Dynamics/Inlet Check Valve ==
  Qs_EHSV : Inport
  Ps : Inport  Port=2
  Divide : Product  Inputs=*/
  EntrappedAir : Constant  Value=ent_air
  Inlet Check Valve Flow : Subsystem
  Integrator : Integrator  InitialCondition=Ps0
  Model : ModelReference  ModelNameDialog=BulkModulus  SimulationMode=Normal  ModelReferenceVersion=1.12  CopyOfModelName=BulkModulus  DefaultDataLogging=on
  Product : Product  RndMeth=Zero
  Sum : Sum  Inputs=-+|
  Temperature : Constant  Value=Temp
  Vcv : Constant  Value=Vcv
  Qs_CV : Outport
  Ps_CV : Outport  Port=2
  wires:
  Inlet Check Valve Flow/1(Q) -> Sum/2, Qs_CV/1
  Qs_EHSV/1 -> Sum/1
  Integrator/1 -> Inlet Check Valve Flow/2(P2), Ps_CV/1
  Sum/1 -> Product/2
  Product/1 -> Integrator/1
  Temperature/1 -> [Temperature]
  EntrappedAir/1 -> [EntrappedAir]
  Ps/1 -> Model/2, Inlet Check Valve Flow/1(P1)
  [Temperature] -> Model/1
  [EntrappedAir] -> Model/3
  Divide/1 -> Product/1
  Model/1 -> Divide/1
  Vcv/1 -> Divide/2

== system RudderActuatorChannel_control_arx/Actuation System/Actuator/Valves Dynamics/Return Check Valve ==
  Pt : Inport
  Qt_EHSV : Inport  Port=2
  Qacv : Inport  Port=3
  Bus Selector1 : BusSelector  OutputSignals=Qacv1,Qacv2
  Divide : Product  Inputs=*/
  EntrappedAir : Constant  Value=ent_air
  Integrator : Integrator  InitialCondition=Pt0
  Model : ModelReference  ModelNameDialog=BulkModulus  SimulationMode=Normal  ModelReferenceVersion=1.12  CopyOfModelName=BulkModulus  DefaultDataLogging=on
  Product : Product  RndMeth=Zero
  Return Check Valve Flow : Subsystem
  Sum : Sum  Inputs=+--
  Sum1 : Sum  Inputs=++|
  Temperature : Constant  Value=Temp
  Vcv : Constant  Value=Vcv
  Pt_CV : Outport
  Qt_CV : Outport  Port=2
  wires:
  Sum/1 -> Product/2
  Integrator/1 -> Return Check Valve Flow/2(P2), Pt_CV/1
  Pt/1 -> Model/2, Return Check Valve Flow/1(P1)
  Qt_EHSV/1 -> Sum/1
  Return Check Valve Flow/1(Q) -> Qt_CV/1, Sum/2
  Product/1 -> Integrator/1
  Qacv/1 -> Bus Selector1/1
  Bus Selector1/1 -> Sum1/1  "<Qacv1>"
  Bus Selector1/2 -> Sum1/2  "<Qacv2>"
  Sum1/1 -> Sum/3
  Temperature/1 -> [Temperature]
  EntrappedAir/1 -> [EntrappedAir]
  [Temperature] -> Model/1
  [EntrappedAir] -> Model/3
  Divide/1 -> Product/1
  Model/1 -> Divide/1
  Vcv/1 -> Divide/2

== system RudderActuatorChannel_control_arx/Actuation System/Electronics System/Analog Controller/Kinematics ==
  ThetaS : Inport
  Constant : Constant  Value=L0
  Constant1 : Constant  Value=R
  Constant2 : Constant  Value=C
  Constant3 : Constant  Value=Theta0
  Law of cosines Get side : Fcn  Expr=sqrt(u(1)^2+u(2)^2-2*u(1)*u(2)*cos(u(3)))
  Mux1 : Mux  Inputs=3
  Sum : Sum  Inputs=|++
  Sum1 : Sum  Inputs=|+-
  Xp : Outport
  wires:
  Constant2/1 -> Mux1/1  "C"
  Constant1/1 -> Mux1/2  "R"
  Mux1/1 -> Law of cosines Get side/1
  ThetaS/1 -> Sum/1  "ThetaS"
  Sum/1 -> Mux1/3
  Law of cosines Get side/1 -> Sum1/1  "L"
  Constant/1 -> Sum1/2  "L0"
  Sum1/1 -> Xp/1
  Constant3/1 -> Sum/2  "Theta0"

== system RudderActuatorChannel_control_arx/Actuation System/Electronics System/Analog Controller/LQR ==
  Ref : Inport
  Xobs : Inport  Port=2
  Add : Sum  Inputs=|+-
  Add1 : Sum  Inputs=|+-
  Demux1 : Demux  Outputs=6
  Gain : Gain  Gain=K(5)
  Gain1 : Gain  Gain=[K(1:4) K(6)]./K(5)  Multiplication=Matrix(K*u) (u vector)
  Mux : Mux  Inputs=5
  u : Outport
  wires:
  Xobs/1 -> Demux1/1
  Demux1/6 -> Mux/5
  Demux1/4 -> Mux/4
  Demux1/3 -> Mux/3
  Demux1/2 -> Mux/2
  Demux1/1 -> Mux/1
  Ref/1 -> Add/1
  Demux1/5 -> Add/2
  Add/1 -> Add1/1
  Mux/1 -> Gain1/1
  Add1/1 -> Gain/1
  Gain/1 -> u/1
  Gain1/1 -> Add1/2

== system RudderActuatorChannel_control_arx/Actuation System/Electronics System/Analog Controller/Reduced order observer ==
  y : Inport
  u : Inport  Port=2
  A : Gain  Gain=A  Multiplication=Matrix(K*u)
  Add : Sum  Inputs=+++
  Add1 : Sum
  Demux : Demux  Outputs=3
  Demux1 : Demux  Outputs=3
  H : Gain  Gain=H  Multiplication=Matrix(K*u)
  Integrator : Integrator
  K : Gain  Gain=K  Multiplication=Matrix(K*u)
  L : Gain  Gain=L  Multiplication=Matrix(K*u)
  Mux : Mux  Inputs=6
  Xobs : Outport
  wires:
  y/1 -> Demux1/1, K/1, L/1
  H/1 -> Add/2
  u/1 -> H/1
  A/1 -> Add/3
  L/1 -> Add/1
  Add/1 -> Integrator/1
  Integrator/1 -> A/1, Add1/2
  K/1 -> Add1/1
  Add1/1 -> Demux/1
  Demux1/1 -> Mux/1
  Demux1/2 -> Mux/4
  Demux1/3 -> Mux/5
  Demux/1 -> Mux/2
  Demux/2 -> Mux/3
  Demux/3 -> Mux/6
  Mux/1 -> Xobs/1

== system RudderActuatorChannel_control_arx/Actuation System/Electronics System/Digital Controller/Kinematics ==
  ThetaS : Inport
  Constant : Constant  Value=L0
  Constant1 : Constant  Value=R
  Constant2 : Constant  Value=C
  Constant3 : Constant  Value=Theta0
  Law of cosines Get side : Fcn  Expr=sqrt(u(1)^2+u(2)^2-2*u(1)*u(2)*cos(u(3)))  SampleTime=T_ES
  Mux1 : Mux  Inputs=3
  Sum : Sum  Inputs=|++  SampleTime=T_ES
  Sum1 : Sum  Inputs=|+-  SampleTime=T_ES
  Xp : Outport
  wires:
  Constant2/1 -> Mux1/1  "C"
  Constant1/1 -> Mux1/2  "R"
  Mux1/1 -> Law of cosines Get side/1
  ThetaS/1 -> Sum/1  "ThetaS"
  Sum/1 -> Mux1/3
  Law of cosines Get side/1 -> Sum1/1  "L"
  Constant/1 -> Sum1/2  "L0"
  Sum1/1 -> Xp/1
  Constant3/1 -> Sum/2  "Theta0"

== system RudderActuatorChannel_control_arx/Actuation System/Electronics System/Digital Controller/LQR ==
  Ref : Inport
  y : Inport  Port=2
  Add : Sum  Inputs=|+-
  Add1 : Sum  Inputs=|+-
  Demux1 : Demux  Outputs=3
  Gain : Gain  Gain=K(3)
  Gain1 : Gain  Gain=[K(1) K(2)]./K(3)  Multiplication=Matrix(K*u) (u vector)
  Input control : Scope  NumInputPorts=2
      settings: TimeRange=1.515675675675676  YMin=-5.9091e-26~-400000  YMax=0.0671053~200000  SaveName=ScopeData6
  Mux : Mux  Inputs=2
  u : Outport
  wires:
  y/1 -> Demux1/1
  Ref/1 -> Add/1
  Add/1 -> Input control/1, Add1/1
  Mux/1 -> Gain1/1
  Add1/1 -> Input control/2, Gain/1
  Gain/1 -> u/1
  Gain1/1 -> Add1/2
  Demux1/1 -> Mux/1
  Demux1/2 -> Mux/2
  Demux1/3 -> Add/2

== system RudderActuatorChannel_control_arx/Actuation System/Electronics System/Digital Controller/PID controller ==
  e : Inport
  Delay : UnitDelay  SampleTime=-1
  Discrete Transfer Fcn : DiscreteTransferFcn  Numerator=[1 1]  Denominator=[1 -1]
  Discrete Transfer Fcn1 : DiscreteTransferFcn  Numerator=[1 1]  Denominator=[1 -1]
  Filter Coefficient1 : Gain  Gain=Ts/2
  Filter Coefficient2 : Gain  Gain=Ki
  Filter Coefficient3 : Gain  Gain=kd_N
  Filter Coefficient4 : Gain  Gain=Ts/2
  Gain : Gain  Gain=Kp
  Gain1 : Gain  Gain=Ki
  Gain2 : Gain  Gain=Kd
  "Saturation " : Saturate  UpperLimit=umax  LowerLimit=-umax  SampleTime=T_ES
  Sum1 : Sum  Inputs=+++
  Sum2 : Sum  Inputs=-+|
  Sum3 : Sum  Inputs=+-
  Sum4 : Sum  Inputs=|+-
  Unit Delay : UnitDelay  SampleTime=-1
  u : Outport
  wires:
  Gain1/1 -> Sum2/2
  Gain/1 -> Sum1/2
  Sum1/1 -> Sum3/1, "Saturation "/1
  e/1 -> Gain2/1, Gain/1, Gain1/1
  Discrete Transfer Fcn/1 -> Sum1/1
  Filter Coefficient1/1 -> Discrete Transfer Fcn/1
  Gain2/1 -> Sum4/1
  Sum2/1 -> Filter Coefficient1/1
  "Saturation "/1 -> u/1, Sum3/2
  Sum3/1 -> Unit Delay/1
  Filter Coefficient2/1 -> Sum2/1
  Unit Delay/1 -> Filter Coefficient2/1
  Sum4/1 -> Filter Coefficient3/1
  Discrete Transfer Fcn1/1 -> Filter Coefficient4/1
  Filter Coefficient4/1 -> Sum4/2
  Delay/1 -> Discrete Transfer Fcn1/1
  Filter Coefficient3/1 -> Sum1/3, Delay/1

== system RudderActuatorChannel_control_arx/Actuation System/Electronics System/Digital Controller/Rate Limit ==
  Cmd : Inport
  Gain : Gain  Gain=1/T_ES
  Gain1 : Gain  Gain=T_ES
  Rate Limit : Saturate  UpperLimit=Rate_Limit  LowerLimit=-Rate_Limit
  Sum3 : Sum  Inputs=|+-  SaturateOnIntegerOverflow=on  InputSameDT=on  OutDataTypeStr=Inherit: Same as first input
  Sum4 : Sum  Inputs=|++  SaturateOnIntegerOverflow=on  InputSameDT=on  OutDataTypeStr=Inherit: Same as first input
  Unit Delay1 : UnitDelay  SampleTime=-1
  Unit Delay2 : UnitDelay  SampleTime=-1
  Cmd_RL : Outport
  wires:
  Cmd/1 -> Sum3/1
  Unit Delay1/1 -> Sum3/2
  Sum3/1 -> Gain/1  "dCmd"
  Gain/1 -> Rate Limit/1  "Rate"
  Rate Limit/1 -> Gain1/1  "Rate Limited"
  Unit Delay2/1 -> Sum4/2
  Sum4/1 -> Unit Delay2/1, Cmd_RL/1, Unit Delay1/1
  Gain1/1 -> Sum4/1

== system RudderActuatorChannel_control_arx/Actuation System/Electronics System/Hardware_in/Signal Processing ==
  Sesnsors_In : Inport
  Add1 : Sum
  Band-Limited White Noise : simulink/Sources/Band-Limited White Noise  Cov=[0.5]  Ts=sampleTime  seed=[23341]
  Bus Creator : BusCreator  Inputs=3
  Bus Selector : BusSelector  OutputSignals=Xp_mesured_(in),dP_mesured_(psi),Xv_mesured_(in)
  RAM LVDT Tolerance : Gain
  Xv LVDT Tolerance : Gain
  dp LVDT Tolerance : Gain
  Sensors_Out : Outport
  wires:
  Sesnsors_In/1 -> Bus Selector/1
  Bus Selector/3 -> Xv LVDT Tolerance/1  "<Xv_mesured_(in)>"
  Bus Selector/1 -> RAM LVDT Tolerance/1  "<Xp_mesured_(in)>"
  Bus Selector/2 -> Add1/1  "<dP_mesured_(psi)>"
  RAM LVDT Tolerance/1 -> Bus Creator/1  "Xp_FB"
  dp LVDT Tolerance/1 -> Bus Creator/2  "dP_FB"
  Xv LVDT Tolerance/1 -> Bus Creator/3  "Xv_FB"
  Bus Creator/1 -> Sensors_Out/1
  Band-Limited White Noise/1 -> Add1/2
  Add1/1 -> dp LVDT Tolerance/1

== system RudderActuatorChannel_control_arx/Actuation System/Actuator/Cylinder Dynamics/Fluid Dynamics/Anti-Cavitation Valve1 ==
  Phigh : Inport
  Plow : Inport  Port=2
  Abs : Abs
  Constant : Constant  Value=Acv*sqrt(2/Rho)
  Constant1 : Constant  Value=Pcvac
  Gain : Gain  Gain=Cd/Pcvac
  Math Function : Math  Operator=sqrt  SaturateOnIntegerOverflow=on
  Product : Product  RndMeth=Zero
  Product1 : Product  RndMeth=Zero
  Product2 : Product  RndMeth=Zero
  Saturation : Saturate  UpperLimit=Cd  LowerLimit=0
  Sign : Signum
  Sum : Sum  Inputs=|+-
  Sum1 : Sum  Inputs=|+-
  Q : Outport
  wires:
  Phigh/1 -> Sum/1
  Plow/1 -> Sum/2
  Sum/1 -> Sum1/1, Abs/1, Sign/1
  Constant1/1 -> Sum1/2
  Sum1/1 -> Gain/1
  Gain/1 -> Saturation/1
  Saturation/1 -> Product/1
  Constant/1 -> Product/2
  Abs/1 -> Math Function/1
  Sign/1 -> Product1/1
  Math Function/1 -> Product1/2
  Product1/1 -> Product2/1
  Product/1 -> Product2/2
  Product2/1 -> Q/1

== system RudderActuatorChannel_control_arx/Actuation System/Actuator/Cylinder Dynamics/Fluid Dynamics/Anti-Cavitation Valve2 ==
  Phigh : Inport
  Plow : Inport  Port=2
  Abs : Abs
  Constant : Constant  Value=Acv*sqrt(2/Rho)
  Constant1 : Constant  Value=Pcvac
  Gain : Gain  Gain=Cd/Pcvac
  Math Function : Math  Operator=sqrt  SaturateOnIntegerOverflow=on
  Product : Product  RndMeth=Zero
  Product1 : Product  RndMeth=Zero
  Product2 : Product  RndMeth=Zero
  Saturation : Saturate  UpperLimit=Cd  LowerLimit=0
  Sign : Signum
  Sum : Sum  Inputs=|+-
  Sum1 : Sum  Inputs=|+-
  Q : Outport
  wires:
  Product2/1 -> Q/1
  Product/1 -> Product2/2
  Product1/1 -> Product2/1
  Math Function/1 -> Product1/2
  Sign/1 -> Product1/1
  Abs/1 -> Math Function/1
  Constant/1 -> Product/2
  Saturation/1 -> Product/1
  Gain/1 -> Saturation/1
  Sum1/1 -> Gain/1
  Constant1/1 -> Sum1/2
  Sum/1 -> Sign/1, Abs/1, Sum1/1
  Plow/1 -> Sum/2
  Phigh/1 -> Sum/1

== system RudderActuatorChannel_control_arx/Actuation System/Actuator/Cylinder Dynamics/Fluid Dynamics/Ext Leak1 ==
  Phigh : Inport
  Plow : Inport  Port=2
  Abs : Abs
  Constant : Constant  Value=Cd*sqrt(2/Rho)
  Constant3 : Constant  Value=Aleakext
  Math Function : Math  Operator=sqrt  SaturateOnIntegerOverflow=on
  Product : Product  RndMeth=Zero
  Product1 : Product  RndMeth=Zero
  Product3 : Product  RndMeth=Zero
  Sign : Signum
  Sum : Sum  Inputs=|+-
  Q : Outport
  wires:
  Phigh/1 -> Sum/1
  Sum/1 -> Abs/1, Sign/1
  Abs/1 -> Math Function/1
  Sign/1 -> Product/1
  Math Function/1 -> Product/2
  Constant/1 -> Product1/2
  Product/1 -> Product1/1
  Constant3/1 -> Product3/2  "Atot"
  Product1/1 -> Product3/1
  Product3/1 -> Q/1
  Plow/1 -> Sum/2

== system RudderActuatorChannel_control_arx/Actuation System/Actuator/Cylinder Dynamics/Fluid Dynamics/Ext Leak2 ==
  Phigh : Inport
  Plow : Inport  Port=2
  Abs : Abs
  Constant : Constant  Value=Cd*sqrt(2/Rho)
  Constant3 : Constant  Value=Aleakext
  Math Function : Math  Operator=sqrt  SaturateOnIntegerOverflow=on
  Product : Product  RndMeth=Zero
  Product1 : Product  RndMeth=Zero
  Product3 : Product  RndMeth=Zero
  Sign : Signum
  Sum : Sum  Inputs=|+-
  Q : Outport
  wires:
  Plow/1 -> Sum/2
  Product3/1 -> Q/1
  Product1/1 -> Product3/1
  Constant3/1 -> Product3/2  "Atot"
  Product/1 -> Product1/1
  Constant/1 -> Product1/2
  Math Function/1 -> Product/2
  Sign/1 -> Product/1
  Abs/1 -> Math Function/1
  Sum/1 -> Sign/1, Abs/1
  Phigh/1 -> Sum/1

== system RudderActuatorChannel_control_arx/Actuation System/Actuator/Cylinder Dynamics/Fluid Dynamics/Int Leak1 ==
  Phigh : Inport
  Plow : Inport  Port=2
  Abs : Abs
  Constant : Constant  Value=Cd*sqrt(2/Rho)
  Constant3 : Constant  Value=Aleakint
  Math Function : Math  Operator=sqrt  SaturateOnIntegerOverflow=on
  Product : Product  RndMeth=Zero
  Product1 : Product  RndMeth=Zero
  Product3 : Product  RndMeth=Zero
  Sign : Signum
  Sum : Sum  Inputs=|+-
  Q : Outport
  wires:
  Plow/1 -> Sum/2
  Product3/1 -> Q/1
  Product1/1 -> Product3/1
  Constant3/1 -> Product3/2  "Atot"
  Product/1 -> Product1/1
  Constant/1 -> Product1/2
  Math Function/1 -> Product/2
  Sign/1 -> Product/1
  Abs/1 -> Math Function/1
  Sum/1 -> Sign/1, Abs/1
  Phigh/1 -> Sum/1

== system RudderActuatorChannel_control_arx/Actuation System/Actuator/Cylinder Dynamics/Fluid Dynamics/Int Leak2 ==
  Phigh : Inport
  Plow : Inport  Port=2
  Abs : Abs
  Constant : Constant  Value=Cd*sqrt(2/Rho)
  Constant3 : Constant  Value=Aleakint
  Math Function : Math  Operator=sqrt  SaturateOnIntegerOverflow=on
  Product : Product  RndMeth=Zero
  Product1 : Product  RndMeth=Zero
  Product3 : Product  RndMeth=Zero
  Sign : Signum
  Sum : Sum  Inputs=|+-
  Q : Outport
  wires:
  Phigh/1 -> Sum/1
  Sum/1 -> Abs/1, Sign/1
  Abs/1 -> Math Function/1
  Sign/1 -> Product/1
  Math Function/1 -> Product/2
  Constant/1 -> Product1/2
  Product/1 -> Product1/1
  Constant3/1 -> Product3/2  "Atot"
  Product1/1 -> Product3/1
  Product3/1 -> Q/1
  Plow/1 -> Sum/2

== system RudderActuatorChannel_control_arx/Actuation System/Actuator/Cylinder Dynamics/Piston Dynamics/Seal Friction Force ==
  Pe : Inport
  Pr : Inport  Port=2
  Xpdot : Inport  Port=3
  Constant : Constant  Value=SealType
  Constant3 : Constant  Value=SealConstValue
  Constant4 : Constant  Value=0
  Force friction 2 Rod backup + scrapper seal : Subsystem
  Force friction Piston+rod extension : Subsystem
  Force friction Piston+rod retraction : Subsystem
  Gain6 : Gain  Gain=Bkp_seal
  Product1 : Product  RndMeth=Zero
  Seal Friction type : MultiPortSwitch
  Stribeck effect : Subsystem
  Sum6 : Sum  Inputs=+++
  FrictionForce_(lbf) : Outport
  wires:
  Constant4/1 -> Force friction 2 Rod backup + scrapper seal/1(Pressure)
  Force friction Piston+rod extension/1(Ffriction) -> Sum6/1
  Force friction Piston+rod retraction/1(Ffriction) -> Sum6/2
  Force friction 2 Rod backup + scrapper seal/1(Ffriction) -> Gain6/1
  Gain6/1 -> Sum6/3
  Pe/1 -> Force friction Piston+rod extension/1(Pressure)
  Pr/1 -> Force friction Piston+rod retraction/1(Pressure)
  Product1/1 -> Seal Friction type/3
  Sum6/1 -> Product1/1, Seal Friction type/2
  Constant/1 -> Seal Friction type/1
  Seal Friction type/1 -> FrictionForce_(lbf)/1
  Constant3/1 -> Seal Friction type/4
  Xpdot/1 -> Stribeck effect/1(Xp)
  Stribeck effect/1(Stribeck factor) -> Product1/2

== system RudderActuatorChannel_control_arx/Actuation System/Actuator/Sensors Dynamics/Xp LVDT /LVDT ==
  Sensor In : Inport
  " Pos Error1" : Lookup_n-D  NumberOfTableDimensions=1  BreakpointsForDimension1=[range(1) range(2) range(3)]  Table=[lvdt_error lvdt_error*0.4 lvdt_error]  RndMeth=Simplest  InputSameDT=on
  Backlash : Backlash  BacklashWidth=(range(3)-range(2))*hyst/100
  LVDT Dynamics1 : TransferFcn  Numerator=[band]  Denominator=[1 band]
  Random1 : RandomNumber  Mean=1  Variance=10
  Sum2 : Sum  Inputs=|++
  Sum3 : Sum  Inputs=|+-
  Switch1 : Switch  Threshold=1
  SensorOut : Outport
  wires:
  [LVDTerror2] -> Sum3/2
  Switch1/1 -> LVDT Dynamics1/1
  Sum2/1 -> Switch1/1
  Sensor In/1 -> Sum2/1, Sum3/1, " Pos Error1"/1
  Random1/1 -> Switch1/2
  [LVDTerror2] -> Sum2/2
  Sum3/1 -> Switch1/3
  " Pos Error1"/1 -> [LVDTerror2]
  LVDT Dynamics1/1 -> Backlash/1
  Backlash/1 -> SensorOut/1

== system RudderActuatorChannel_control_arx/Actuation System/Actuator/Sensors Dynamics/Xv LVDT /LVDT1 ==
  Sensor In : Inport
  " Pos Error1" : Lookup_n-D  NumberOfTableDimensions=1  BreakpointsForDimension1=[range(1) range(2) range(3)]  Table=[lvdt_error lvdt_error*0.4 lvdt_error]  RndMeth=Simplest  InputSameDT=on
  Backlash : Backlash  BacklashWidth=(range(3)-range(2))*hyst/100
  LVDT Dynamics1 : TransferFcn  Numerator=[band]  Denominator=[1 band]
  Random1 : RandomNumber  Mean=1  Variance=10
  Sum2 : Sum  Inputs=|++
  Sum3 : Sum  Inputs=|+-
  Switch1 : Switch  Threshold=1
  SensorOut : Outport
  wires:
  [LVDTerror2] -> Sum3/2
  Switch1/1 -> LVDT Dynamics1/1
  Sum2/1 -> Switch1/1
  Sensor In/1 -> Sum2/1, Sum3/1, " Pos Error1"/1
  Random1/1 -> Switch1/2
  [LVDTerror2] -> Sum2/2
  Sum3/1 -> Switch1/3
  " Pos Error1"/1 -> [LVDTerror2]
  LVDT Dynamics1/1 -> Backlash/1
  Backlash/1 -> SensorOut/1

== system RudderActuatorChannel_control_arx/Actuation System/Actuator/Sensors Dynamics/dP LVDT /LVDT1 ==
  Sensor In : Inport
  " Pos Error1" : Lookup_n-D  NumberOfTableDimensions=1  BreakpointsForDimension1=[range(1) range(2) range(3)]  Table=[lvdt_error lvdt_error*0.4 lvdt_error]  RndMeth=Simplest  InputSameDT=on
  Backlash : Backlash  BacklashWidth=(range(3)-range(2))*hyst/100
  LVDT Dynamics1 : TransferFcn  Numerator=[band]  Denominator=[1 band]
  Random1 : RandomNumber  Mean=1  Variance=10
  Sum2 : Sum  Inputs=|++
  Sum3 : Sum  Inputs=|+-
  Switch1 : Switch  Threshold=1
  SensorOut : Outport
  wires:
  [LVDTerror2] -> Sum3/2
  Switch1/1 -> LVDT Dynamics1/1
  Sum2/1 -> Switch1/1
  Sensor In/1 -> Sum2/1, Sum3/1, " Pos Error1"/1
  Random1/1 -> Switch1/2
  [LVDTerror2] -> Sum2/2
  Sum3/1 -> Switch1/3
  " Pos Error1"/1 -> [LVDTerror2]
  LVDT Dynamics1/1 -> Backlash/1
  Backlash/1 -> SensorOut/1
